simulink model "untitled"  (Simulink 10.0)
settings: Solver=VariableStepAuto  StartTime=0.0  StopTime=10.0  RelTol=1e-3
settings Model: Creator=win_10  LastModifiedBy=win_10
settings DataIOCC: SaveFormat=Dataset  ReturnWorkspaceOutputs=on
settings OptimizationCC: LifeSpan=auto
settings DebuggingCC: UnderspecifiedInitializationDetection=Simplified  MergeDetectMultiDrivingBlocksExec=error  SFUnexpectedBacktrackingDiag=error  SFNoUnconditionalDefaultTransitionDiag=error  SFExecutionAtInitializationDiag=warning  ArithmeticOperatorsInVariantConditions=error
settings HardwareCC: ProdBitPerPointer=64  ProdBitPerSizeT=64  ProdBitPerPtrDiffT=64  ProdLargestAtomicFloat=Float  ProdIntDivRoundTo=Zero  ProdEndianess=LittleEndian  ProdWordSize=64  ProdHWDeviceType=Intel->x86-64 (Windows64)
settings ModelReferenceCC: PropagateSignalLabelsOutOfModel=on
settings SFSimCC: SimUseLocalCustomCode=on  CustomCodeUndefinedFunction=FilterOut
settings RTWCC: RTWUseLocalCustomCode=on
settings CodeAppCC: StateflowObjectComments=off
settings GRTTargetCC: TargetLangStandard=C99 (ISO)  CombineOutputUpdateFcns=on  GRTInterface=off
settings ConfigComp: CovMetricSettings=dwe  CovHtmlReporting=off  CovSaveCumulativeToWorkspaceVar=off  CovSaveSingleToWorkspaceVar=off

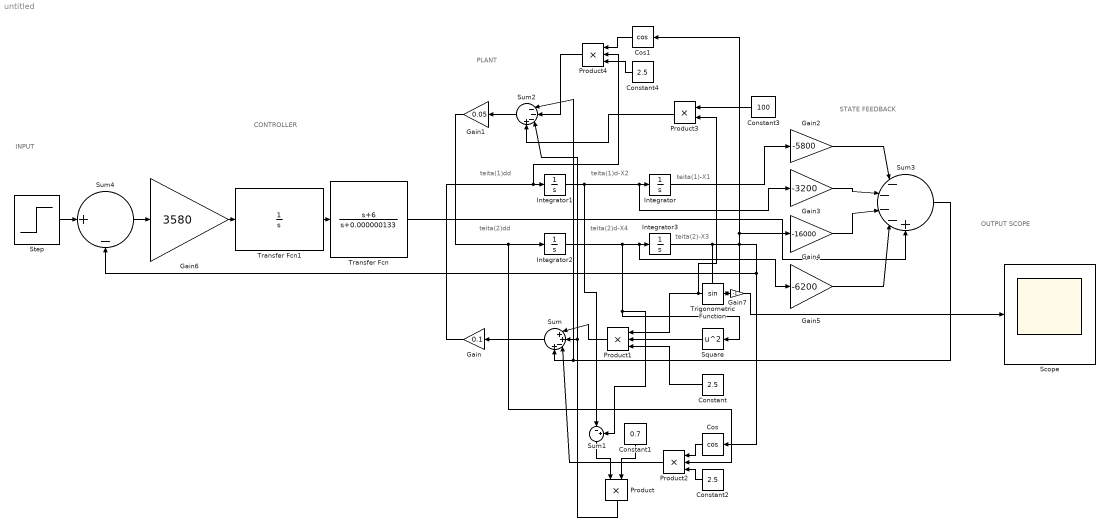
== system untitled ==
  note: INPUT
  note: OUTPUT SCOPE
  note: STATE FEEDBACK
  note: CONTROLLER
  note: PLANT
  note: teita(1)d-X2
  note: teita(2)d-X4
  note: teita(2)-X3
  note: teita(1)dd
  note: teita(2)dd
  note: teita(1)-X1
  Constant : Constant  Value=2.5
  Constant1 : Constant  Value=0.7
  Constant2 : Constant  Value=2.5
  Constant3 : Constant  Value=100
  Constant4 : Constant  Value=2.5
  Cos : Trigonometry  Operator=cos
  Cos1 : Trigonometry  Operator=cos
  Gain : Gain  Gain=0.1
  Gain1 : Gain  Gain=0.05
  Gain2 : Gain  Gain=-5800
  Gain3 : Gain  Gain=-3200
  Gain4 : Gain  Gain=-16000
  Gain5 : Gain  Gain=-6200
  Gain6 : Gain  Gain=3580
  Gain7 : Gain  Gain=-1
  Integrator{,1..3} (4 alike) : Integrator
  Product : Product
  Product1 : Product  Inputs=3
  Product2 : Product  Inputs=3
  Product3 : Product
  Product4 : Product  Inputs=3
  Scope : Scope
  Square : Math  Operator=square  SignedPower=off  SaturateOnIntegerOverflow=on
  Step : Step  Time=0  SampleTime=0
  Sum : Sum  Inputs=|++-+
  Sum1 : Sum  Inputs=|-+
  Sum2 : Sum  Inputs=|---+
  Sum3 : Sum  Inputs=|----+
  Sum4 : Sum  Inputs=|+-
  Transfer Fcn : TransferFcn  Numerator=[1 6]  Denominator=[1 0.000000133]
  Transfer Fcn1 : TransferFcn  Denominator=[1 0]
  Trigonometric Function : Trigonometry
  wires:
  Integrator2/1 -> Square/1, Sum1/2, Gain5/1, Integrator3/1
  Integrator1/1 -> Gain3/1, Integrator/1, Sum1/1
  Integrator3/1 -> Cos1/1, Gain4/1, Sum4/2, Cos/1, Trigonometric Function/1, Gain7/1
  Square/1 -> Product1/2
  Trigonometric Function/1 -> Product3/2, Product1/1
  Constant/1 -> Product1/3
  Product1/1 -> Sum/1
  Constant1/1 -> Product/2
  Sum1/1 -> Product/1
  Product/1 -> Sum2/3, Sum/2
  Gain1/1 -> Product2/2, Integrator2/1
  Cos/1 -> Product2/1
  Constant2/1 -> Product2/3
  Product2/1 -> Sum/3
  Sum/1 -> Gain/1
  Gain/1 -> Product4/2, Integrator1/1
  Sum2/1 -> Gain1/1
  Constant3/1 -> Product3/1
  Product3/1 -> Sum2/4
  Cos1/1 -> Product4/1
  Constant4/1 -> Product4/3
  Product4/1 -> Sum2/2
  Integrator/1 -> Gain2/1
  Gain2/1 -> Sum3/1
  Gain3/1 -> Sum3/2
  Gain4/1 -> Sum3/3
  Gain5/1 -> Sum3/4
  Sum3/1 -> Sum/4, Sum2/1
  Transfer Fcn/1 -> Sum3/5
  Sum4/1 -> Gain6/1
  Step/1 -> Sum4/1
  Transfer Fcn1/1 -> Transfer Fcn/1
  Gain6/1 -> Transfer Fcn1/1
  Gain7/1 -> Scope/1
